simulink model "simulink_find_corr"  (R2016a)
settings: Solver=VariableStepAuto  StartTime=0.0  StopTime=inf  RelTol=1e-3
model workspace (MAT data in the model file):
  Param = Simulink.Parameter
  Param.DataType = 'auto'
  Param.Dimensions = [0 0]
  Var = 0
libraries: audiosources x1, dspstat3 x1, dspsrcs4 x1
settings Model: Creator=Hongji  LastModifiedBy=Hongji

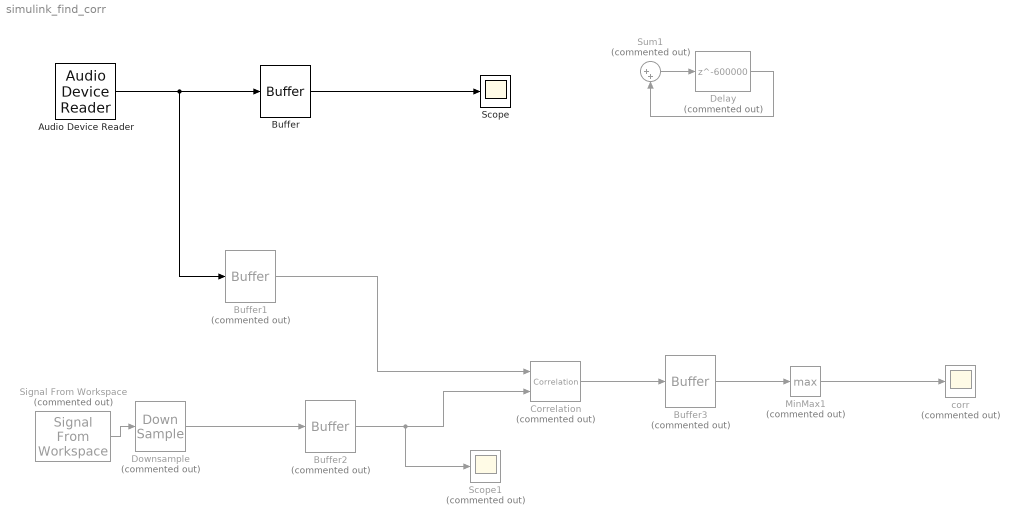
== system simulink_find_corr ==
  Audio Device Reader : audiosources/Audio Device Reader  Driver=DirectSound  Device=Microphone (High Definition Audio Device)  SampleRate=200000  NumChannels=1  SamplesPerFrame=400  BitDepth=16-bit integer  NumBuffers=10  DefaultInputChannelMapping=on  InputChannelMapping=1:2  OutputNumOverrunSamples=off  OutputDataType=double  DriverIdx=1  DeviceWarnFlag=''
  Buffer : Buffer  N=1  TreatMby1Signals=One channel  OutputFrames=off
  Buffer1 : Buffer  Commented=on  N=1500  TreatMby1Signals=One channel  OutputFrames=off
  Buffer2 : Buffer  Commented=on  N=1500  TreatMby1Signals=One channel  OutputFrames=off
  Buffer3 : Buffer  Commented=on  N=100  TreatMby1Signals=One channel  OutputFrames=off
  Correlation : dspstat3/Correlation  Commented=on  domain=Frequency  outputDataTypeStr=Inherit: Same as accumulator  outputLastDataTypeStr=Inherit: Same as accumulator  outputMin=[]  outputMax=[]  roundingMode=Floor  overflowMode=off
  Delay : Delay  Commented=on  DelayLength=600000  InputProcessing=Columns as channels (frame based)
  Downsample : DownSample  Commented=on  N=100
  MinMax1 : MinMax  Commented=on  Function=max  ZeroCross=off
  Scope : Scope
  Scope1 : Scope  Commented=on
  Signal From Workspace : dspsrcs4/Signal From Workspace  Commented=on  X=precise_claps  Ts=1/200000  nsamps=150000  OutputAfterFinalValue=Cyclic repetition  ignoreOrWarnInputAndFrameLengths=off  OutputFrames=off
  Sum1 : Sum  Commented=on  Inputs=|++
  "corr " : Scope  Commented=on
  wires:
  Audio Device Reader/1 -> Buffer1/1, Buffer/1
  Delay/1 -> Sum1/2
  Sum1/1 -> Delay/1
  Buffer/1 -> Scope/1
  Buffer1/1 -> Correlation/1
  Signal From Workspace/1 -> Downsample/1
  Downsample/1 -> Buffer2/1
  Buffer2/1 -> Scope1/1, Correlation/2
  Correlation/1 -> Buffer3/1
  Buffer3/1 -> MinMax1/1
  MinMax1/1 -> "corr "/1
